simulink model "cw5_model_BORKOWSKI_17"  (R2017b)
settings: Solver=VariableStepAuto  StartTime=0.0  StopTime=10.0  MaxStep=0.01  MinStep=0.001  RelTol=1e-6
undefined symbols (not defined in the file): A, a0, a1, B, b0, C, D
settings Model: Creator=Student  LastModifiedBy=Kamil
settings DataIOCC: SaveFormat=Array
settings DebuggingCC: UnconnectedInputMsg=none  UnconnectedOutputMsg=none  UnconnectedLineMsg=none
settings ModelReferenceCC: EnableRefExpFcnMdlSchedulingChecks=off
settings SFSimCC: SimUseLocalCustomCode=on
settings RTWCC: Description=Generic Real-Time Target  RTWUseLocalCustomCode=on
settings CodeAppCC: StateflowObjectComments=on

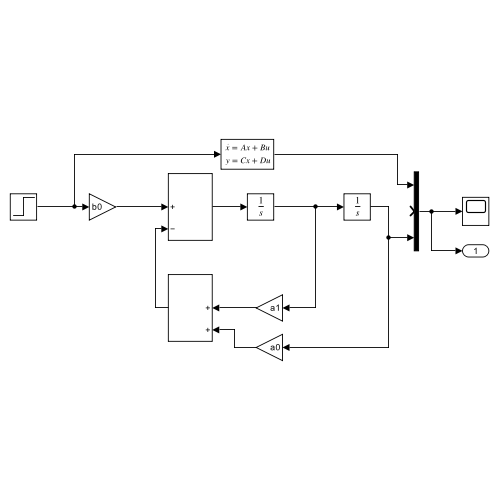
[thumbnail: Simulink's stored preview of the top-level diagram]
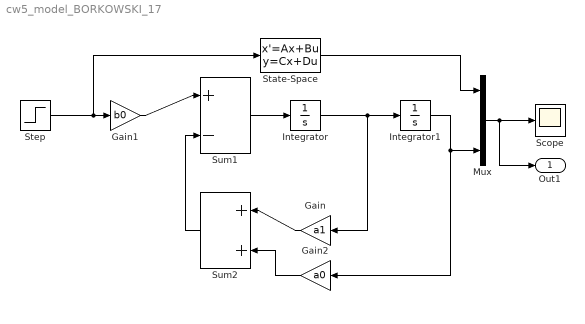
== system cw5_model_BORKOWSKI_17 ==
  Gain : Gain  Gain=a1
  Gain1 : Gain  Gain=b0
  Gain2 : Gain  Gain=a0
  Integrator : Integrator
  Integrator1 : Integrator
  Mux : Mux  Inputs=3
  Scope : Scope
  State-Space : StateSpace  A=A  B=B  C=C  D=D  InitialCondition=0
  Step : Step  Time=0  Before=1  SampleTime=0
  Sum1 : Sum  Inputs=|+-
  Sum2 : Sum  Inputs=|++
  Out1 : Outport
  wires:
  Mux/1 -> Out1/1, Scope/1
  Integrator1/1 -> Gain2/1, Mux/3
  Integrator/1 -> Gain/1, Integrator1/1
  Sum1/1 -> Integrator/1
  Gain1/1 -> Sum1/1
  Step/1 -> State-Space/1, Gain1/1
  Sum2/1 -> Sum1/2
  Gain/1 -> Sum2/1
  Gain2/1 -> Sum2/2
  State-Space/1 -> Mux/1
